simulink model "RBNN_NNT_timing_of_learning_1layerRBNN"  (R2019a)
settings: Solver=FixedStepAuto  StartTime=0.0  StopTime=inf  FixedStep=0.000001  RelTol=1e-3
libraries: dspstat3 x6, dspxfrm3 x1
(part 1 of 3)
settings Model: NumberOfSteps=3200  Creator=vardhah  LastModifiedBy=vardhah
settings DataIOCC: ReturnWorkspaceOutputs=off
settings DebuggingCC: UnderSpecifiedDimensionMsg=warning  ArithmeticOperatorsInVariantConditions=warning

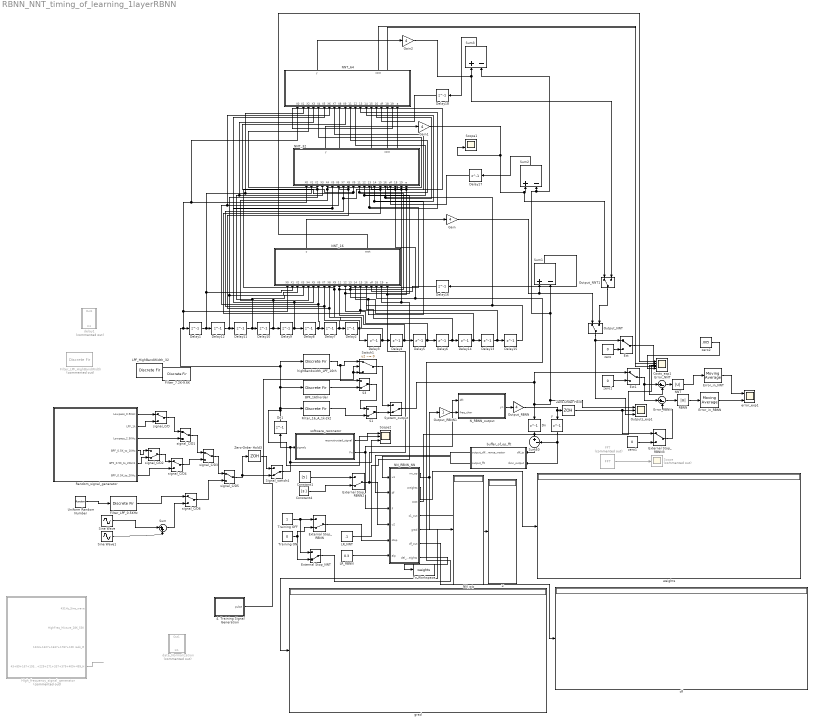
== system RBNN_NNT_timing_of_learning_1layerRBNN ==
  4. Training Signal Generation : MATLAB Function  TreatAsAtomicUnit=on
  BPF_16thorder : DiscreteFir  Tag=BlockMethodSubSystem  Coefficients=[-0.0560788660629819163 -0.080220031928137342 -0.085169812197034192 -0.0616477005407154097 -0.0104987832754634518 0.0560691321297696263 0.118166811935027122 0.155549755804414214 0.155549755804414214 0.118166811935027122 0.0560691321297696263 -0.0104987832754634518 -0.0616477005407154097 -0.085169812197034192 -0.080220031928137342 -0.0560788660629819163]  InputProcessing=Columns as channels (frame based)  SampleTime=0.0001
  Constant1 : Constant  Value=[5 ]
  Constant4 : Constant  Value=[3 ]
  Costs_exp1 : Scope  NumInputPorts=5
  Delay{1..18} (18 alike) : Delay  DelayLength=1  InitialCondition=0
  Dn : Delay  DelayLength=1  InitialCondition=0
  Dn1 : Delay  DelayLength=1  InitialCondition=0
  Error_NNT : Sum  Inputs=|+-
  Error_RBNN : Sum  Inputs=|+-
  Error_in_NNT : dspstat3/Moving Average  Method=Sliding window  ForgettingFactorPort=off  SpecifyWindowLength=on  WindowLength=32  ForgettingFactor=0.9  SimulateUsing=Code generation
  Error_in_RBNN : dspstat3/Moving Average  Method=Sliding window  ForgettingFactorPort=off  SpecifyWindowLength=on  WindowLength=32  ForgettingFactor=0.9  SimulateUsing=Code generation
  Ext : ManualSwitch
  Ext1 : ManualSwitch
  External Stop_NNT : ManualSwitch  CurrentSetting=0
  External Stop_RBNN : ManualSwitch  CurrentSetting=0
  External Stop_RBNN2 : ManualSwitch  CurrentSetting=0
  External Stop_RBNN3 : ManualSwitch
  FFT : dspxfrm3/FFT  Commented=on  FFTImplementation=Auto  CompMethod=Table lookup  TableOpt=NEW  TableOptActive=Speed  BitRevOrder=off  Normalize=off  InheritFFTLength=off  FFTLength=16  WrapInput=on  roundingMode=Floor  overflowMode=off  firstCoeffDataTypeStr=Inherit: Same word length as input  firstCoeffLastDataTypeStr=Inherit: Same word length as input  outputMin=[]  outputMax=[]
  Filter_16_A_1k-2k2 : DiscreteFir  Tag=BlockMethodSubSystem  Coefficients=[-0.198889914644374777 0.0882189428518377339 0.0736891495871065116 0.0638368801789635787 0.0566372642221577294 0.0523172683654103132 0.0494565343907736044 0.048157521822162791 0.048157521822162791 0.0494565343907736044 0.0523172683654103132 0.0566372642221577294 0.0638368801789635787 0.0736891495871065116 0.0882189428518377339 -0.198889914644374777]  InputProcessing=Columns as channels (frame based)  SampleTime=0.0001
  "Filter_7.2K-9.6K " : DiscreteFir  Tag=BlockMethodSubSystem  Coefficients=[-0.0120785049852322399 -0.0942455273574688279 0.0101245004695954266 0.125460404555770566 0.034165372769331126 -0.1614987160724079 -0.0984930555982914957 0.150982315564688691 0.150982315564688691 -0.0984930555982914957 -0.1614987160724079 0.034165372769331126 0.125460404555770566 0.0101245004695954266 -0.0942455273574688279 -0.0120785049852322399]  InputProcessing=Columns as channels (frame based)  SampleTime=0.0001
  Filter_LPF_0.5KHz : DiscreteFir  Tag=BlockMethodSubSystem  Coefficients=[-3.18896299597288383e-06 -3.83354529240465071e-06 -4.05165684067063815e-06 -3.70503419237271275e-06 -2.71906990921963897e-06 -1.10676148924612755e-06 1.01752303220119839e-06 3.43816546660442561e-06 5.85432915205445393e-06 7.91172475253303529e-06 9.24748198063262036e-06 9.54314441329317781e-06 8.57891464218529322e-06 6.28119063306686426e-06 2.75540703838948166e-06 -1.70264685833682874e-06 -6.62155398741489909e-06 -1.13963160872715597e-05 -1.53551787741418131e-05 -1.78448003404143785e-05 -1.83239149312040147e-05 -1.64532505445185763e-05 -1.2168551650234288e-05 -5.72441542640661863e-06 2.30065286328061826e-06 1.10432130014885979e-05 1.94375819130544083e-05 2.63358228239397591e-05 3.06527409547321919e-05 3.15188143471818768e-05 2.84210704759463182e-05 2.13114557654784512e-05 1.06645441623202335e-05 -2.52855191172796634e-06 -1.68358930597779849e-05 -3.05270440995195151e-05 -4.17697383326380358e-05 -4.88600682263782041e-05 -5.04588674894021949e-05 -4.58034816997138439e-05 -3.48644674245972617e-05 -1.84212146734814604e-05 1.96117233985991472e-06 2.40599458870630971e-05 4.52206320563785464e-05 6.26601296191042951e-05 7.38143039151016979e-05 7.66886373067194368e-05 7.01664557973317001e-05 5.4230853663410808e-05 3.0063946604706336e-05 -9.06910547433990952e-19 -3.2673952472505879e-05 -6.40570677143264015e-05 -9.00810854331069799e-05 -0.000107015428312995711 -0.000111970713168571331 -0.000103335721558068123 -8.10862895771685482e-05 -4.69162356045351654e-05 -4.15947022375518983e-06 4.25030843521332388e-05 8.75309599149356896e-05 0.000125158632964597209 0.000150107231853438973 0.000158288513539332098 0.0001474108253235409 0.000117402630625484597 7.0586296289757748e-05 1.15618160619801507e-05 -5.32057851390989819e-05 -0.000116064331613017162 -0.000169050673564196974 -0.000204868252016619302 -0.000217849502697044413 -0.000204780400830474336 -0.000165473493715557389 -0.000102999876487308575 -2.35276731508314631e-05 6.42391728862500407e-05 0.000149977898849883878 0.000222927980880206121 0.0002732051725498416 0.000293092128479146815 0.000278142039348765505 0.000227944728914647769 0.000146437518782008096 4.16929407521120276e-05 -7.48231683727459198e-05 -0.000189463559059635484 -0.000287959140544256096 -0.000357152780500302421 -0.000386701420546690228 -0.000370532032329052164 -0.000307854784659617809 -0.000203580374088952956 -6.80538327357860825e-05 8.39026635588222257e-05 0.000234559610599040989 0.000365303187296817577 0.000458886227964114366 0.000501640477869142939 0.000485372957627082098 0.000408692778022271387 0.00027757124940440078 0.000105022400798701802 -9.01059221851134746e-05 -0.000285130206460953181 -0.000456114886506772807 -0.000580753711624647489 -0.000641208429359311225 -0.000626551095678341916 -0.000534486311946431392 -0.000372101500347091403 -0.000155500252257189596 9.16956221899910116e-05 0.000340850438698926542 0.000561569363925951701 0.000725341273075596755 0.000809140607016507014 0.000798541886443339356 0.000689937687510389823 0.000491540555242624935 0.000222983084508023412 -8.65061031602710578e-05 -0.000401198257171604233 -0.000682915574655691931 -0.000895587169454724222 -0.00100977497122057614 -0.00100661170820988714 -0.000880637893554398637 -0.000641134931496952073 -0.000311716673629381465 7.18557261654923163e-05 0.000465454153269549253 0.000821572791381306637 0.00109497291918021398 0.00124832280526836594 0.00125714126766055738 0.00111340594095754629 0.000827320717287859954 0.000426938590774311277 -4.44153582223980888e-05 -0.000532709198051358542 -0.000979292567766554571 -0.00132783509343295156 -0.00153130628952159275 -0.00155814589516756327 -0.00139683328419227854 -0.00105822385340401961 -0.000575264157102420184 8.51170167667764168e-18 0.000601881631178106057 0.00115842388311454916 0.00159987308294497546 0.00186727082204797925 0.00192012343287634862 0.00174217269081196379 0.00134447901059969776 0.000765320349639572826 6.67755071975156323e-05 -0.000671741772575677049 -0.00136234854839730433 -0.0019189880490347159 ...(+8051 chars)]  InputProcessing=Columns as channels (frame based)  SampleTime=0.0001
  Filter_LPF_HighBandWidth : DiscreteFir  Tag=BlockMethodSubSystem  Commented=on  Coefficients=[0.00257561197553052117 0.0149226993015543988 -0.0126813197622564593 0.0131583623867790739 -0.0109438145213804211 0.00462377218068549256 0.00574880781840408916 -0.0188595701191665473 0.032156879848246514 -0.042054633169390801 0.0443249918452583783 -0.0343435917303160365 0.00670297923827019304 0.0478068572768818173 -0.160206703181909604 0.618531838092966302 0.618531838092966302 -0.160206703181909604 0.0478068572768818173 0.00670297923827019304 -0.0343435917303160365 0.0443249918452583783 -0.042054633169390801 0.032156879848246514 -0.0188595701191665473 0.00574880781840408916 0.00462377218068549256 -0.0109438145213804211 0.0131583623867790739 -0.0126813197622564593 0.0149226993015543988 0.00257561197553052117]  InputProcessing=Columns as channels (frame based)  SampleTime=0.0001
  Gain : Gain  Gain=4
  Gain1 : Gain  Gain=4
  Gain2 : Gain  Gain=4
  HIgh_frequency_signal_generator : Subsystem  Commented=on
  LPF_HighBandWidth_32 : DiscreteFir  Tag=BlockMethodSubSystem  Coefficients=[0.00257561197553052117 0.0149226993015543988 -0.0126813197622564593 0.0131583623867790739 -0.0109438145213804211 0.00462377218068549256 0.00574880781840408916 -0.0188595701191665473 0.032156879848246514 -0.042054633169390801 0.0443249918452583783 -0.0343435917303160365 0.00670297923827019304 0.0478068572768818173 -0.160206703181909604 0.618531838092966302 0.618531838092966302 -0.160206703181909604 0.0478068572768818173 0.00670297923827019304 -0.0343435917303160365 0.0443249918452583783 -0.042054633169390801 0.032156879848246514 -0.0188595701191665473 0.00574880781840408916 0.00462377218068549256 -0.0109438145213804211 0.0131583623867790739 -0.0126813197622564593 0.0149226993015543988 0.00257561197553052117]  InputProcessing=Columns as channels (frame based)  SampleTime=0.0001
  LR_NNT : Constant  Value=.1
  LR_RBNN : Constant  Value=0.3
  NNT : Abs
  NNT_16 : MATLAB Function  TreatAsAtomicUnit=on  SystemSampleTime=0.0001
  NNT_32 : MATLAB Function  TreatAsAtomicUnit=on  SystemSampleTime=0.0001
  NNT_64 : MATLAB Function  TreatAsAtomicUnit=on  SystemSampleTime=0.0001
  NN_RBNN_NN : MATLAB Function  TreatAsAtomicUnit=on
  NN_o/p : Display
  N_RBNN_output : MATLAB Function  TreatAsAtomicUnit=on
  Output_NNT : ManualSwitch
  Output_NNT1 : ManualSwitch
  Output_RBNN : Gain  Gain=4
  Output_RBNN1 : Gain
  Outputs_exp1 : Scope  NumInputPorts=3
  RBNN : Abs
  Random_signal_generator : Subsystem
  S1 : ManualSwitch  CurrentSetting=0
  S3 : ManualSwitch  CurrentSetting=0
  Scope : Scope  Commented=on
  Scope1 : Scope  NumInputPorts=2
  Scope2 : Scope  NumInputPorts=3
  Signal_switch4 : ManualSwitch  CurrentSetting=0
  Sine Wave : Sin  Frequency=139  SampleTime=0.0001
  Sine Wave1 : Sin  Frequency=557  SampleTime=0.0001
  Sum : Sum  Inputs=|++
  Sum1 : Sum  Inputs=+-
  Sum2 : Sum  Inputs=+-
  Sum3 : Sum  Inputs=+-
  Sum50 : Sum  Inputs=|+-
  Switch1 : Switch  Criteria=u2 ~= 0
  "System_output " : ManualSwitch  CurrentSetting=0
  To Workspace : ToWorkspace  VariableName=weights  SaveFormat=Timeseries  SampleTime=-1
  Training OFF : Constant
  Training ON : Constant  Value=0
  Uniform Random Number : UniformRandomNumber  SampleTime=0.000001
  Z : Display
  Zero-Order Hold : ZeroOrderHold  SampleTime=-1
  Zero-Order Hold3 : ZeroOrderHold  SampleTime=0.0001
  buffer_of_op_fft : MATLAB Function  TreatAsAtomicUnit=on
  data_Normalization : Subsystem  Commented=on
  delay1 : Subsystem  Commented=on
  df : Display
  error_exp1 : Scope  NumInputPorts=2
  grad : Display
  highBandwidth_LPF_16th : DiscreteFir  Tag=BlockMethodSubSystem  Coefficients=[-0.0297618438739734592 -0.0348768570143923456 0.0417652636536197108 0.0516071256815222451 -0.0669316025800295866 -0.0943151588376726635 0.157872597041064711 0.474640475929861472 0.474640475929861472 0.157872597041064711 -0.0943151588376726635 -0.0669316025800295866 0.0516071256815222451 0.0417652636536197108 -0.0348768570143923456 -0.0297618438739734592]  InputProcessing=Columns as channels (frame based)  SampleTime=0.0001
  signal_C/D{,1,3..6} (6 alike) : ManualSwitch
  signal_C/D2 : ManualSwitch  CurrentSetting=0
  software_rezonator : MATLAB Function  TreatAsAtomicUnit=on  SystemSampleTime=0.0001
  weights : Display
  y : Delay  DelayLength=1  InitialCondition=0
  zero : Constant  Value=0
  zero1 : Constant  Value=0
  "zero1 " : Constant  Value=0
  zero2 : Constant  Value=.005
  wires:
  software_rezonator/1(reconstructed_signal) -> Scope2/1
  software_rezonator/2(Fn) -> NN_RBNN_NN/3(F), N_RBNN_output/1(dft)
  N_RBNN_output/1(yn) -> Output_RBNN/1
  Dn/1 -> Sum50/1
  y/1 -> buffer_of_op_fft/2(rbnn_output), Sum50/2
  NN_RBNN_NN/1(nn_op) -> NN_o/p/1, Output_RBNN1/1
  Training OFF/1 -> External Stop_NNT/1, External Stop_RBNN/1
  Training ON/1 -> External Stop_NNT/2, External Stop_RBNN/2
  NN_RBNN_NN/3(cost) -> Costs_exp1/3
  NN_RBNN_NN/2(weights) -> weights/1
  NN_RBNN_NN/4(z1_out) -> Z/1
  Sum50/1 -> buffer_of_op_fft/1(dif_ip)
  buffer_of_op_fft/1(output_difference_vector) -> NN_RBNN_NN/2(df)
  buffer_of_op_fft/2(output_fft) -> NN_RBNN_NN/1(u1)
  NNT_16/1(y) -> Gain/1
  Delay16/1 -> NNT_16/17(df)
  Delay4/1 -> NNT_32/11(X10), NNT_64/11(X10), NNT_16/11(X10), Delay5/1
  Delay6/1 -> Delay14/1, NNT_32/13(X12), NNT_64/13(X12), NNT_16/13(X12)
  Delay5/1 -> NNT_32/12(X11), NNT_64/12(X11), NNT_16/12(X11), Delay6/1
  NNT_16/2(cost) -> Costs_exp1/1
  Delay2/1 -> Delay3/1, NNT_64/9(X8), NNT_32/9(X8), NNT_16/9(X8)
  Delay15/1 -> NNT_32/16(X15), NNT_64/16(X15), NNT_16/16(X15)
  Delay13/1 -> NNT_16/15(X14), NNT_64/15(X14), NNT_32/15(X14), Delay15/1
  Delay14/1 -> NNT_32/14(X13), NNT_64/14(X13), NNT_16/14(X13), Delay13/1
  Delay10/1 -> NNT_16/5(X4), NNT_64/5(X4), NNT_32/5(X4), Delay9/1
  signal_C/D5/1 -> Zero-Order Hold3/1, Signal_switch4/2
  Delay3/1 -> Delay4/1, NNT_32/10(X9), NNT_64/10(X9), NNT_16/10(X9)
  Delay7/1 -> Delay2/1, NNT_32/8(X7), NNT_64/8(X7), NNT_16/8(X7)
  Delay8/1 -> NNT_32/7(X6), NNT_64/7(X6), NNT_16/7(X6), Delay7/1
  Delay1/1 -> NNT_64/2(X1), NNT_32/2(X1), NNT_16/2(X1), Delay12/1
  Delay9/1 -> Delay8/1, NNT_16/6(X5), NNT_32/6(X5), NNT_64/6(X5)
  Delay12/1 -> NNT_64/3(X2), NNT_32/3(X2), NNT_16/3(X2), Delay11/1
  Delay11/1 -> Delay10/1, NNT_32/4(X3), NNT_64/4(X3), NNT_16/4(X3)
  Sum1/1 -> Delay16/1
  Error_RBNN/1 -> RBNN/1
  Error_NNT/1 -> NNT/1
  Gain/1 -> Output_NNT/1, Sum1/1
  LR_RBNN/1 -> NN_RBNN_NN/6(alp)
  RBNN/1 -> Error_in_RBNN/1
  NNT/1 -> Error_in_NNT/1
  Error_in_NNT/1 -> error_exp1/1
  Error_in_RBNN/1 -> error_exp1/2
  External Stop_NNT/1 -> NNT_64/18(stop), NNT_32/18(stop), NNT_16/18(stop)
  Output_RBNN/1 -> y/1, Zero-Order Hold/1
  LR_NNT/1 -> NNT_64/19(alpha_l), NNT_32/19(alpha_l), NNT_16/19(alpha_l)
  HIgh_frequency_signal_generator/4(43+89+167+193+229+271+337+379+409+499_H) -> ?
  Zero-Order Hold3/1 -> Signal_switch4/1
  FFT/1 -> Scope/1
  Switch1/1 -> "System_output "/1
  Constant1/1 -> External Stop_RBNN2/1
  4. Training Signal Generation/1(pulse) -> Switch1/3, Switch1/2
  Constant4/1 -> External Stop_RBNN2/2
  External Stop_RBNN2/1 -> NNT_64/20(a), NNT_32/20(a), NNT_16/20(a), NN_RBNN_NN/4(u2)
  NNT_32/1(y) -> Gain1/1
  Gain1/1 -> Scope1/2, Output_NNT1/1, Sum2/1
  Sum2/1 -> Delay17/1
  Delay17/1 -> NNT_32/17(df)
  Output_NNT/1 -> Outputs_exp1/3, Ext/1
  BPF_16thorder/1 -> S3/2
  S3/1 -> S1/1
  S1/1 -> "System_output "/2
  highBandwidth_LPF_16th/1 -> S3/1, Switch1/1
  Output_RBNN1/1 -> N_RBNN_output/2(freq_char)
  NN_RBNN_NN/5(grad) -> grad/1
  Zero-Order Hold/1 -> External Stop_RBNN3/1, Outputs_exp1/2
  NN_RBNN_NN/6(df_out) -> df/1
  "System_output "/1 -> Ext1/1, Dn/1, Sum3/2, Sum2/2, Sum1/2, Outputs_exp1/1
  NN_RBNN_NN/7(del_weights) -> To Workspace/1
  Signal_switch4/1 -> Scope2/3, Dn1/1, software_rezonator/1(signalz)
  signal_C/D/1 -> signal_C/D1/1
  Random_signal_generator/3(Lowpass_2.5KHz) -> signal_C/D1/2
  Random_signal_generator/4(BPF_0.5K_to_1KHz) -> signal_C/D2/1
  signal_C/D3/1 -> signal_C/D5/1
  signal_C/D1/1 -> signal_C/D3/1
  Random_signal_generator/1(Lowpass_0.5KHz) -> signal_C/D/1
  Random_signal_generator/2(LPF_1k) -> signal_C/D/2
  "zero1 "/1 -> External Stop_RBNN3/2
  External Stop_RBNN3/1 -> Error_RBNN/2
  Ext/1 -> Error_NNT/2
  zero/1 -> Ext/2
  zero1/1 -> Ext1/2
  Ext1/1 -> Error_RBNN/1, Error_NNT/1
  zero2/1 -> Costs_exp1/5
  Random_signal_generator/5(BPF_0.5K_to_2KHz1) -> signal_C/D2/2
  signal_C/D2/1 -> signal_C/D4/1
  Random_signal_generator/6(BPF_0.5K_to_2KHz) -> signal_C/D4/2
  signal_C/D4/1 -> signal_C/D3/2
  Sum3/1 -> Delay18/1
  Delay18/1 -> NNT_64/17(df)
  NNT_64/1(y) -> Gain2/1
  Gain2/1 -> Output_NNT1/2, Sum3/1
  Output_NNT1/1 -> Output_NNT/2
  External Stop_RBNN/1 -> NN_RBNN_NN/5(stop)
  NNT_32/2(cost) -> Costs_exp1/2
  NNT_64/2(cost) -> Costs_exp1/4
  Dn1/1 -> Filter_16_A_1k-2k2/1, BPF_16thorder/1, highBandwidth_LPF_16th/1, NNT_64/1(X0), NNT_32/1(X0), NNT_16/1(X0), Delay1/1, Scope2/2
  Sine Wave/1 -> Sum/1
  Sine Wave1/1 -> Sum/2
  Uniform Random Number/1 -> Filter_LPF_0.5KHz/1
  Filter_LPF_0.5KHz/1 -> signal_C/D6/1
  Sum/1 -> signal_C/D6/2
  signal_C/D6/1 -> signal_C/D5/2
  Filter_16_A_1k-2k2/1 -> S1/2

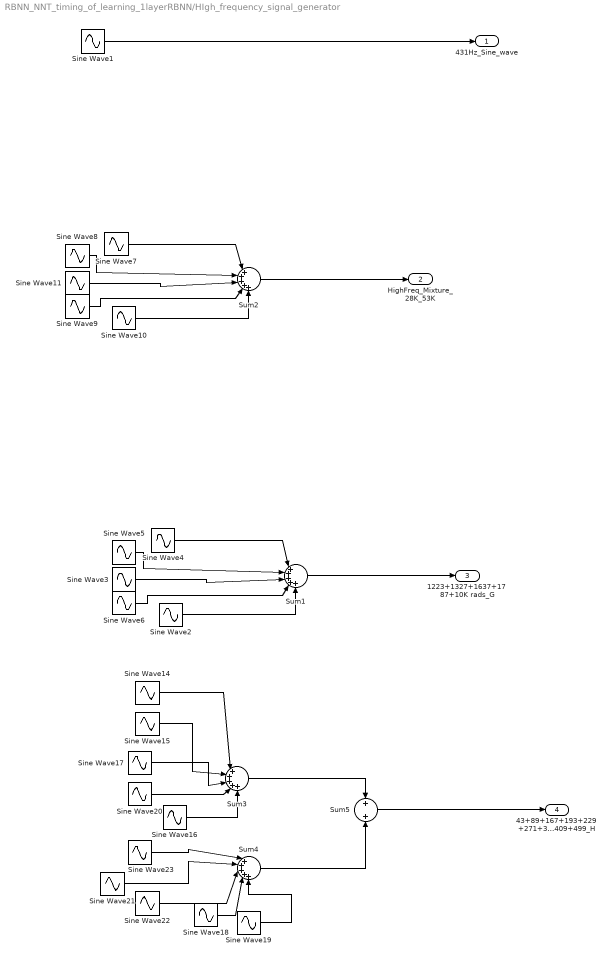
== system RBNN_NNT_timing_of_learning_1layerRBNN/HIgh_frequency_signal_generator ==
  Sine Wave1 : Sin  Amplitude=0.5  Frequency=23000  SampleTime=0.0001
  Sine Wave10 : Sin  Amplitude=0.5  Frequency=7000  SampleTime=0
  Sine Wave11 : Sin  Amplitude=2  Frequency=3637  SampleTime=0
  Sine Wave14 : Sin  Amplitude=0.1  Frequency=43  SampleTime=0
  Sine Wave15 : Sin  Amplitude=0.1  Frequency=89  SampleTime=0
  Sine Wave16 : Sin  Amplitude=0.1  Frequency=229  SampleTime=0
  Sine Wave17 : Sin  Amplitude=0.1  Frequency=167  SampleTime=0
  Sine Wave18 : Sin  Amplitude=0.1  Frequency=409  SampleTime=0
  Sine Wave19 : Sin  Amplitude=0.1  Frequency=499  SampleTime=0
  Sine Wave2 : Sin  Amplitude=0  Frequency=5000  SampleTime=0
  Sine Wave20 : Sin  Amplitude=0.1  Frequency=193  SampleTime=0
  Sine Wave21 : Sin  Amplitude=0.1  Frequency=337  SampleTime=0
  Sine Wave22 : Sin  Amplitude=0.1  Frequency=379  SampleTime=0
  Sine Wave23 : Sin  Amplitude=0.1  Frequency=271  SampleTime=0
  Sine Wave3 : Sin  Amplitude=0.25  Frequency=200  SampleTime=0
  Sine Wave4 : Sin  Amplitude=0.25  Frequency=50  SampleTime=0
  Sine Wave5 : Sin  Amplitude=0.25  Frequency=100  SampleTime=0
  Sine Wave6 : Sin  Amplitude=0.25  Frequency=1787  SampleTime=0
  Sine Wave7 : Sin  Amplitude=2  Frequency=2230  SampleTime=0
  Sine Wave8 : Sin  Amplitude=2  Frequency=5927  SampleTime=0
  Sine Wave9 : Sin  Amplitude=2  Frequency=3787  SampleTime=0
  Sum{1..4} (4 alike) : Sum  Inputs=|+++++
  Sum5 : Sum
  431Hz_Sine_wave : Outport
  HighFreq_Mixture_28K_53K : Outport  Port=2
  1223+1327+1637+1787+10K rads_G : Outport  Port=3
  43+89+167+193+229+271+337+379+409+499_H : Outport  Port=4
  wires:
  Sine Wave9/1 -> Sum2/4
  Sine Wave7/1 -> Sum2/1
  Sine Wave10/1 -> Sum2/5
  Sine Wave8/1 -> Sum2/2
  Sine Wave11/1 -> Sum2/3
  Sum2/1 -> HighFreq_Mixture_28K_53K/1
  Sine Wave23/1 -> Sum4/1
  Sine Wave17/1 -> Sum3/3
  Sine Wave22/1 -> Sum4/3
  Sine Wave18/1 -> Sum4/4
  Sine Wave19/1 -> Sum4/5
  Sine Wave5/1 -> Sum1/2
  Sine Wave20/1 -> Sum3/4
  Sine Wave4/1 -> Sum1/1
  Sine Wave14/1 -> Sum3/1
  Sine Wave15/1 -> Sum3/2
  Sine Wave21/1 -> Sum4/2
  Sine Wave16/1 -> Sum3/5
  Sine Wave6/1 -> Sum1/4
  Sum4/1 -> Sum5/2
  Sum3/1 -> Sum5/1
  Sine Wave2/1 -> Sum1/5
  Sine Wave3/1 -> Sum1/3
  Sum1/1 -> 1223+1327+1637+1787+10K rads_G/1
  Sum5/1 -> 43+89+167+193+229+271+337+379+409+499_H/1
  Sine Wave1/1 -> 431Hz_Sine_wave/1
